simulink model "dc_motor_simulink"  (R2021b)
settings: Solver=VariableStepAuto  StartTime=0.0  StopTime=30  RelTol=1e-3
libraries: simulink x3, fuzblock x1
settings Model: Creator=pappa  LastModifiedBy=pappa

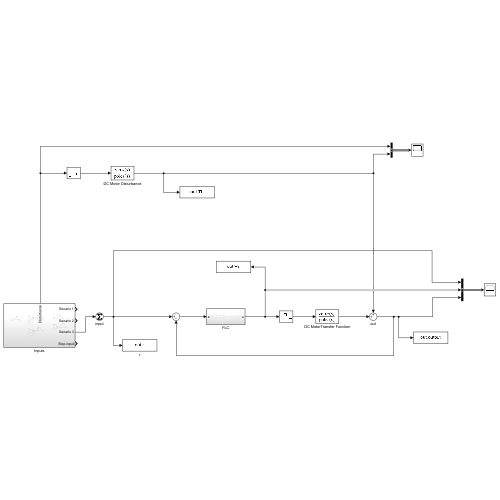
[thumbnail: Simulink's stored preview of the top-level diagram]
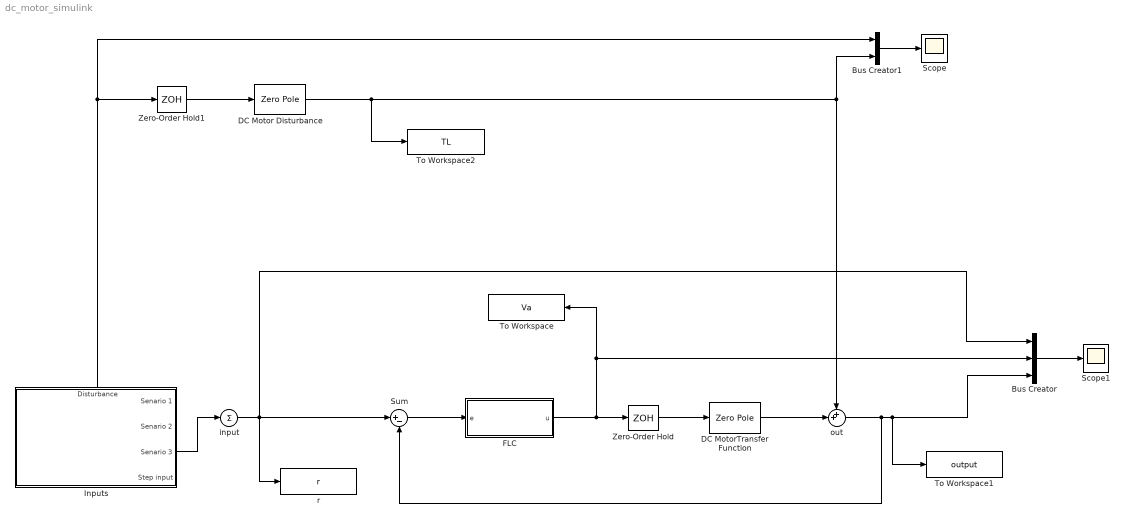
== system dc_motor_simulink ==
  Bus Creator : BusCreator  Inputs=3
  Bus Creator1 : BusCreator  Inputs=2
  DC Motor Disturbance : ZeroPole  Zeros=[-440]  Poles=[-12.064]  Gain=[-2.92]
  DC MotorTransfer Function : ZeroPole  Zeros=[]  Poles=[-12.064]  Gain=[18.69]
  FLC : Subsystem
  Inputs : Subsystem
      settings: PortSchema="{\"entries\":[{\"content\":{\"sides\":[{\"content\":{\"connectorIds\":[]},\"type\":\"ConnectorPlacement.EquallySpacedRectSide\",\"uuid\":\"e5d037f7-dd4b-4110-bc6c-2b9518a2722d\"},{\"content\":{\"connectorIds\":[\"Out1\",\"Out2\",\"Out3\",\"Out4\"],\"side\":\"RIGHT\"},\"type\":\"ConnectorPlacement.EquallySpacedRectSide\",\"uuid\":\"e6e4a1ff-09b4-4b15-8bbf-fa7b3445026f\"},{\"content\":{\"connectorIds\":[\"Out5\"],\"side\":\"TOP\"},\"type\":\"ConnectorPlacement.EquallySpacedRectSide\",\"uuid\":\"c7cd5e8d-a396-416e-bdec-432e5e409340\"}]},\"type\":\"ConnectorPlacement.EquallySpacedConnector\",\"uuid\":\"ef83825a-f63e-4898-88f1-6bb620bd4fed\"}],\"packageUris\":[\"http://schema.mathworks.com/mf0/Connector/R2020b\"],\"version\":\"1.0\"}"
  Scope : Scope
  Scope1 : Scope
  Sum : Sum  Inputs=|+-
  To Workspace : ToWorkspace  VariableName=Va  SaveFormat=Timeseries  SampleTime=0.01
  To Workspace1 : ToWorkspace  VariableName=output  SaveFormat=Timeseries  SampleTime=0.01
  To Workspace2 : ToWorkspace  VariableName=TL  SaveFormat=Timeseries  SampleTime=-1
  Zero-Order Hold : ZeroOrderHold  SampleTime=0.01
  Zero-Order Hold1 : ZeroOrderHold  SampleTime=0.01
  input : Sum  Inputs=+
  out : Sum  Inputs=++|
  r : ToWorkspace  VariableName=r  SaveFormat=Timeseries  SampleTime=0.01
  wires:
  Sum/1 -> FLC/1(e)
  FLC/1(u) -> Bus Creator/2, To Workspace/1, Zero-Order Hold/1
  Zero-Order Hold/1 -> DC MotorTransfer Function/1
  Bus Creator/1 -> Scope1/1
  input/1 -> Bus Creator/1, r/1, Sum/1
  Inputs/5(Disturbance) -> Bus Creator1/1, Zero-Order Hold1/1
  DC MotorTransfer Function/1 -> out/2
  out/1 -> Sum/2, Bus Creator/3, To Workspace1/1
  DC Motor Disturbance/1 -> To Workspace2/1, Bus Creator1/2, out/1
  Zero-Order Hold1/1 -> DC Motor Disturbance/1
  Bus Creator1/1 -> Scope/1
  Inputs/3(Senario 3) -> input/1

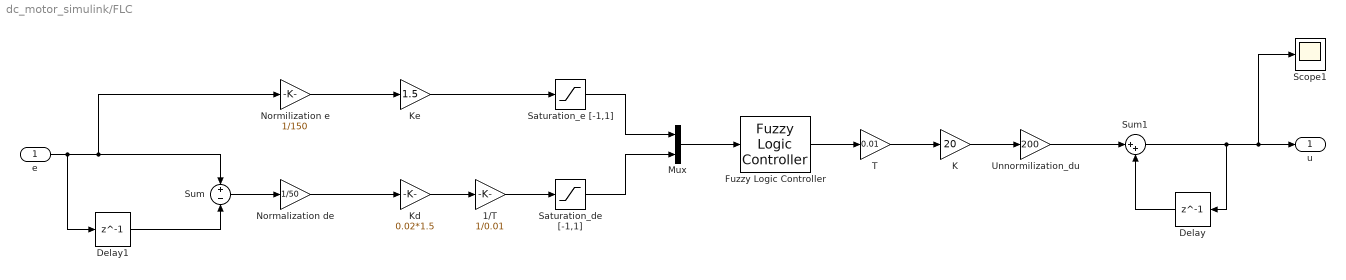
== system dc_motor_simulink/FLC ==
  e : Inport
  1/T : Gain  Gain=1/0.01
  Delay : Delay  DelayLength=1  InitialCondition=0  SampleTime=0.01
  Delay1 : Delay  DelayLength=1  InitialCondition=0  SampleTime=0.01
  Fuzzy Logic Controller : fuzblock/Fuzzy Logic  Controller  FIS='fuzzy_pi.fis'  OutputSampleNumber=101  DataType=double  FuzzifiedInputs=off  RuleFiringStrengths=off  RuleOutputs=off  AggregatedOutputs=off  SimulateUsing=Interpreted execution  OutOfRangeInputValueMessage=warning  NoRuleFiredMessage=warning  EmptyOutputFuzzySetMessage=warning
  K : Gain  Gain=20
  Kd : Gain  Gain=0.02*1.5
  Ke : Gain  Gain=1.5
  Mux : Mux  Inputs=2
  Normalization de : Gain  Gain=1/50
  Normilization e : Gain  Gain=1/150
  Saturation_de [-1,1] : Saturate  UpperLimit=1  LowerLimit=-1
  Saturation_e [-1,1] : Saturate  UpperLimit=1  LowerLimit=-1
  Scope1 : Scope
  Sum : Sum  Inputs=+-
  Sum1 : Sum  Inputs=|++
  T : Gain  Gain=0.01
  Unnormilization_du : Gain  Gain=200
  u : Outport
  wires:
  Unnormilization_du/1 -> Sum1/1
  Ke/1 -> Saturation_e [-1,1]/1
  Saturation_e [-1,1]/1 -> Mux/1
  e/1 -> Delay1/1, Normilization e/1, Sum/1
  Sum1/1 -> Delay/1, Scope1/1, u/1
  Kd/1 -> 1/T/1
  K/1 -> Unnormilization_du/1
  Fuzzy Logic Controller/1 -> T/1
  Saturation_de [-1,1]/1 -> Mux/2
  Mux/1 -> Fuzzy Logic Controller/1
  T/1 -> K/1
  1/T/1 -> Saturation_de [-1,1]/1
  Delay/1 -> Sum1/2
  Sum/1 -> Normalization de/1
  Delay1/1 -> Sum/2
  Normilization e/1 -> Ke/1
  Normalization de/1 -> Kd/1

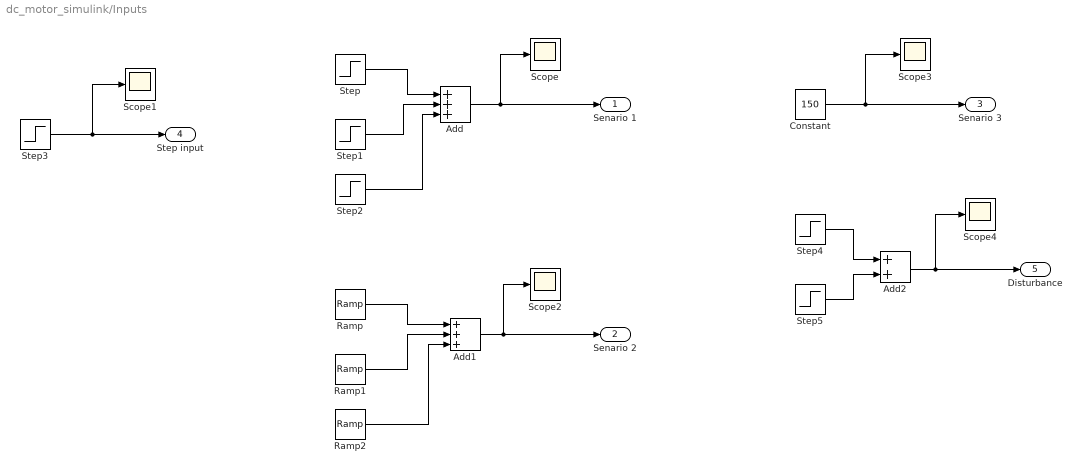
== system dc_motor_simulink/Inputs ==
  Add : Sum  Inputs=+++
  Add1 : Sum  Inputs=+++
  Add2 : Sum
  Constant : Constant  Value=150  SampleTime=0.01
  Ramp : simulink/Sources/Ramp  slope=15  start=0  InitialOutput=0
  Ramp1 : simulink/Sources/Ramp  slope=-15  start=10  InitialOutput=0
  Ramp2 : simulink/Sources/Ramp  slope=-15  start=20  InitialOutput=0
  Scope{,1..4} (5 alike) : Scope
  Step : Step  Time=0  Before=150  After=150  SampleTime=0.01
  Step1 : Step  Time=10  After=-50  SampleTime=0.01
  Step2 : Step  Time=20  After=50  SampleTime=0.01
  Step3 : Step  Time=0  After=150  SampleTime=0.01
  Step4 : Step  Time=10  SampleTime=0.01
  Step5 : Step  Time=20  After=-0.5  SampleTime=0.01
  Senario 1 : Outport
  Senario 2 : Outport  Port=2
  Senario 3 : Outport  Port=3
  Step input : Outport  Port=4
  Disturbance : Outport  Port=5
  wires:
  Step1/1 -> Add/2
  Step2/1 -> Add/3
  Add/1 -> Senario 1/1, Scope/1
  Step/1 -> Add/1
  Step3/1 -> Scope1/1, Step input/1
  Add1/1 -> Scope2/1, Senario 2/1
  Ramp/1 -> Add1/1
  Ramp1/1 -> Add1/2
  Ramp2/1 -> Add1/3
  Constant/1 -> Scope3/1, Senario 3/1
  Step4/1 -> Add2/1
  Step5/1 -> Add2/2
  Add2/1 -> Scope4/1, Disturbance/1
